simulink model "questao2"  (R2021b)
settings: Solver=VariableStepAuto  StartTime=0.0  StopTime=1800  RelTol=1e-3
values from neighbouring files (symbols this model uses):
  A = [A11 A12 ... (first row only)    [main.m]
  B = [Bu Bd]    [main.m]
  C = [1 0]    [main.m]
  D = zeros(1,4)    [main.m]
  dF = 0    [main.m]
  dFj = 4.72e-5    (= 4.72e-05)    [main.m]
  dTi = 0    [main.m]
  dTij = 0    [main.m]
  Ts = 51.67    [main.m]
settings Model: Creator=luang  LastModifiedBy=luang

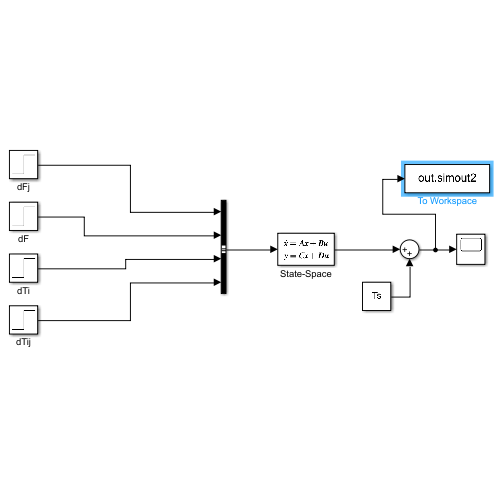
[thumbnail: Simulink's stored preview of the top-level diagram]
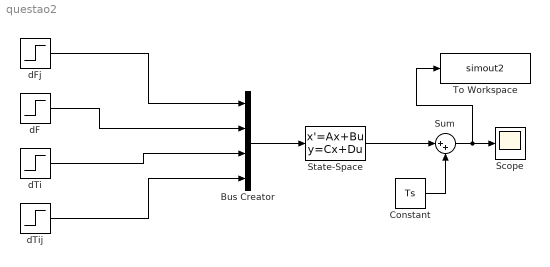
== system questao2 ==
  Bus Creator : BusCreator  Inputs=4
  Constant : Constant  Value=Ts
  Scope : Scope
  State-Space : StateSpace  A=A  B=B  C=C  D=D  InitialCondition=0
  Sum : Sum  Inputs=|++
  To Workspace : ToWorkspace  VariableName=simout2  SaveFormat=Structure With Time  SampleTime=-1
  dF : Step  After=dF  SampleTime=0
  dFj : Step  After=dFj  SampleTime=0
  dTi : Step  After=dTi  SampleTime=0
  dTij : Step  After=dTij  SampleTime=0
  wires:
  Bus Creator/1 -> State-Space/1
  dFj/1 -> Bus Creator/1
  dF/1 -> Bus Creator/2
  dTi/1 -> Bus Creator/3
  dTij/1 -> Bus Creator/4
  State-Space/1 -> Sum/1
  Constant/1 -> Sum/2
  Sum/1 -> To Workspace/1, Scope/1
